simulink subsystem "rss_AgEvalModeCalcNeed"  (R2023a)
settings: Solver=VariableStepAuto  StartTime=0.0  StopTime=10.0  RelTol=1e-3
settings Model: Creator=xiaoqiang.yuan  LastModifiedBy=xiaoqiang.yuan

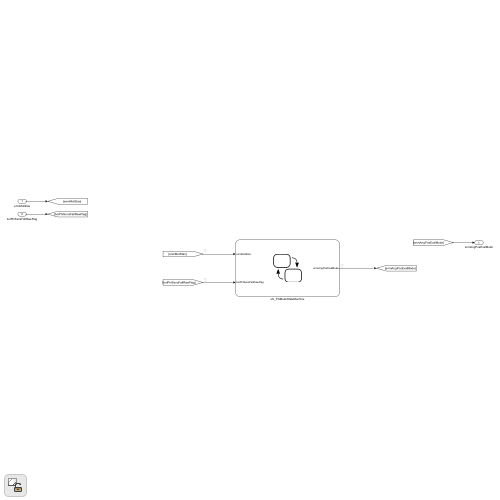
[thumbnail: Simulink's stored preview of the top-level diagram]
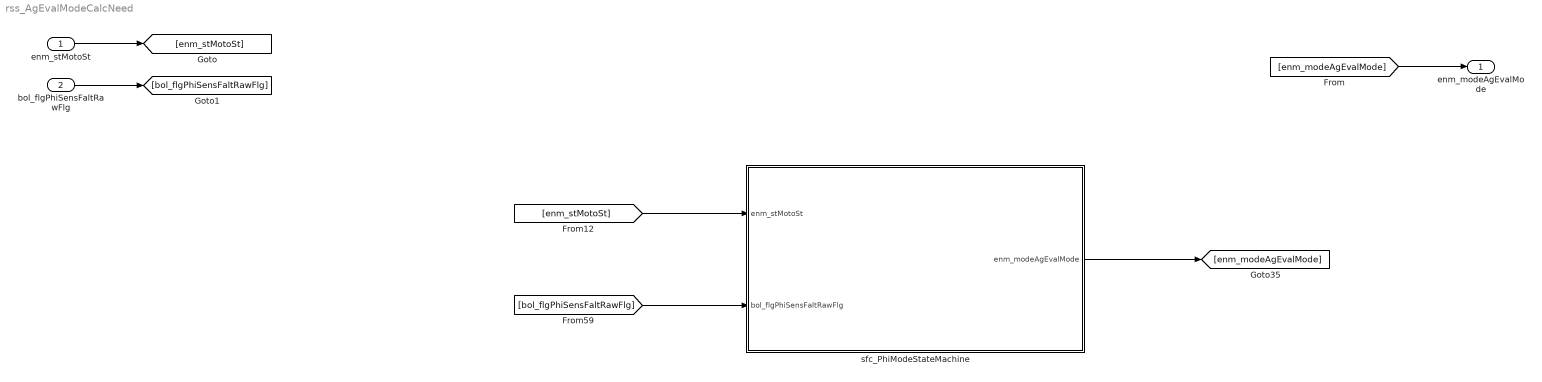
== system rss_AgEvalModeCalcNeed ==
  enm_stMotoSt : Inport  OutDataTypeStr=Enum: ENM_MOTO_STATUS
  bol_flgPhiSensFaltRawFlg : Inport  Port=2  OutDataTypeStr=boolean
  sfc_PhiModeStateMachine : Stateflow chart  TreatAsAtomicUnit=on
  enm_modeAgEvalMode : Outport
  wires:
  [enm_modeAgEvalMode] -> enm_modeAgEvalMode/1
  [enm_stMotoSt] -> sfc_PhiModeStateMachine/1(enm_stMotoSt)
  sfc_PhiModeStateMachine/1(enm_modeAgEvalMode) -> [enm_modeAgEvalMode]
  enm_stMotoSt/1 -> [enm_stMotoSt]
  [bol_flgPhiSensFaltRawFlg] -> sfc_PhiModeStateMachine/2(bol_flgPhiSensFaltRawFlg)
  bol_flgPhiSensFaltRawFlg/1 -> [bol_flgPhiSensFaltRawFlg]

== stateflow chart rss_AgEvalModeCalcNeed/sfc_PhiModeStateMachine ==
  state SENSOR
    en:
    enm_modeAgEvalMode =ENM_AG_POS_EVAL_MODE.SENSOR;
  state SENSORLESS
    en:
    enm_modeAgEvalMode =ENM_AG_POS_EVAL_MODE.SENSORLESS;
  state HYBRID
    en:
    enm_modeAgEvalMode =ENM_AG_POS_EVAL_MODE.HYBRID;
  (default) -> SENSOR
  SENSOR -> SENSORLESS [order 2] : [(enm_stMotoSt == ENM_MOTO_STATUS.OFF && bol_flgPhiSensFaltRawFlg) ||...
      | Genm_modeAgEvallMode_C ==ENM_AG_POS_EVAL_MODE.SENSORLESS]
  SENSORLESS -> SENSOR [order 1] : [Genm_modeAgEvallMode_C == ENM_AG_POS_EVAL_MODE.SENSOR &&...
      | ~bol_flgPhiSensFaltRawFlg]
  HYBRID -> SENSOR [order 1] : [Genm_modeAgEvallMode_C == ENM_AG_POS_EVAL_MODE.SENSOR]
  SENSOR -> HYBRID [order 1] : [Genm_modeAgEvallMode_C == ENM_AG_POS_EVAL_MODE.HYBRID]
  SENSORLESS -> HYBRID [order 2] : [Genm_modeAgEvallMode_C == ENM_AG_POS_EVAL_MODE.HYBRID &&...
      | ~bol_flgPhiSensFaltRawFlg]
  HYBRID -> SENSORLESS [order 2] : [(enm_stMotoSt == ENM_MOTO_STATUS.OFF && bol_flgPhiSensFaltRawFlg) ||...
      | Genm_modeAgEvallMode_C == ENM_AG_POS_EVAL_MODE.SENSORLESS]
  data: Genm_modeAgEvallMode_C parameter; enm_modeAgEvalMode output Enum: ENM_AG_POS_EVAL_MODE; enm_stMotoSt input Enum: ENM_MOTO_STATUS; bol_flgPhiSensFaltRawFlg input boolean
